simulink library "hysteresis_rods"  (R2016b)
settings: Solver=VariableStepAuto  StartTime=0.0  StopTime=10.0  RelTol=1e-3
undefined symbols (not defined in the file or in its folder): sim_params
libraries: aerolibutil x1
settings Model: Creator=Sean  LastModifiedBy=bijan

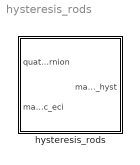
== system hysteresis_rods ==
  hysteresis_rods : Subsystem

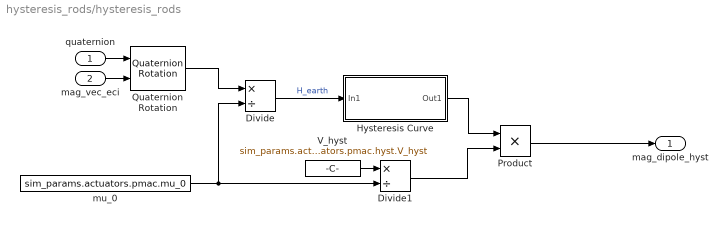
== system hysteresis_rods/hysteresis_rods ==
  quaternion : Inport
  mag_vec_eci : Inport  Port=2
  Divide : Product  Inputs=*/
  Divide1 : Product  Inputs=*/
  Hysteresis Curve : Subsystem
  Product : Product
  Quaternion Rotation : aerolibutil/Quaternion Rotation
  V_hyst : Constant  Value=sim_params.actuators.pmac.hyst.V_hyst
  mu_0 : Constant  Value=sim_params.actuators.pmac.mu_0
  mag_dipole_hyst : Outport
  wires:
  quaternion/1 -> Quaternion Rotation/1
  mag_vec_eci/1 -> Quaternion Rotation/2
  mu_0/1 -> Divide1/2, Divide/2
  Quaternion Rotation/1 -> Divide/1
  Divide/1 -> Hysteresis Curve/1(In1)  "H_earth"
  V_hyst/1 -> Divide1/1
  Hysteresis Curve/1(Out1) -> Product/1
  Divide1/1 -> Product/2
  Product/1 -> mag_dipole_hyst/1

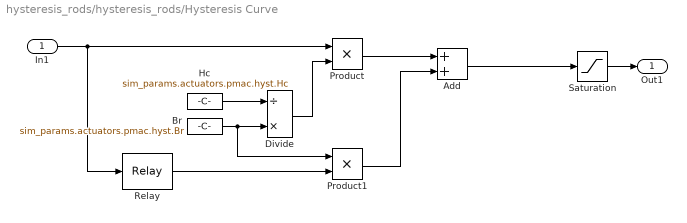
== system hysteresis_rods/hysteresis_rods/Hysteresis Curve ==
  In1 : Inport
  Add : Sum
  Br : Constant  Value=sim_params.actuators.pmac.hyst.Br
  Divide : Product  Inputs=/*
  Hc : Constant  Value=sim_params.actuators.pmac.hyst.Hc
  Product : Product
  Product1 : Product
  Relay : Relay  OnSwitchValue=sim_params.actuators.pmac.on  OffSwitchValue=sim_params.actuators.pmac.off  OffOutputValue=-1
  Saturation : Saturate  UpperLimit=sim_params.actuators.pmac.hyst.Bs  LowerLimit=-sim_params.actuators.pmac.hyst.Bs
  Out1 : Outport
  wires:
  Br/1 -> Product1/1, Divide/2
  Divide/1 -> Product/2
  In1/1 -> Product/1, Relay/1
  Saturation/1 -> Out1/1
  Product/1 -> Add/1
  Hc/1 -> Divide/1
  Relay/1 -> Product1/2
  Product1/1 -> Add/2
  Add/1 -> Saturation/1
